simulink model "teme2eci_test"  (R2018b)
settings: Solver=VariableStepAuto  StartTime=0.0  StopTime=10.0  RelTol=1e-3
libraries: teme2eci_lib x1, time_Lib x1
settings Model: Creator=Kate  LastModifiedBy=Kate

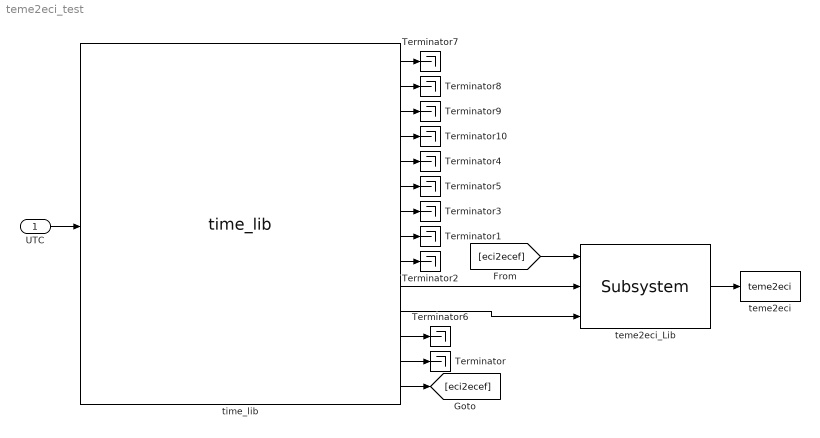
== system teme2eci_test ==
  UTC : Inport
  Terminator{,1..10} (11 alike) : Terminator
  teme2eci : ToWorkspace  VariableName=teme2eci  SampleTime=-1
      settings: Save2DSignal=2-D array (concatenate along first dimension)
  teme2eci_Lib : teme2eci_lib/Subsystem  SystemSampleTime=-1
  "time_lib " : time_Lib/time_lib    SystemSampleTime=-1
  wires:
  "time_lib "/11 -> teme2eci_Lib/3
  "time_lib "/10 -> teme2eci_Lib/2
  "time_lib "/14 -> [eci2ecef]
  [eci2ecef] -> teme2eci_Lib/1
  "time_lib "/13 -> Terminator/1
  "time_lib "/12 -> Terminator6/1
  "time_lib "/9 -> Terminator2/1
  "time_lib "/8 -> Terminator1/1
  "time_lib "/7 -> Terminator3/1
  "time_lib "/6 -> Terminator5/1
  "time_lib "/5 -> Terminator4/1
  "time_lib "/4 -> Terminator10/1
  "time_lib "/3 -> Terminator9/1
  "time_lib "/2 -> Terminator8/1
  "time_lib "/1 -> Terminator7/1
  UTC/1 -> "time_lib "/1
  teme2eci_Lib/1 -> teme2eci/1
